simulink library "sl_nmea"  (R2017b)
settings: Solver=VariableStepAuto  StartTime=0.0  StopTime=10.0  RelTol=1e-3
settings Model: Creator=Bre  LastModifiedBy=bb6223s

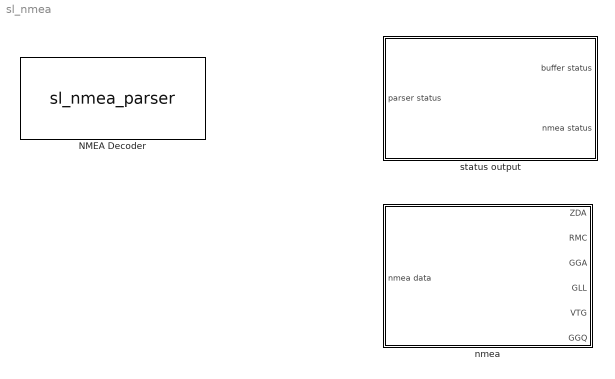
== system sl_nmea ==
  NMEA Decoder : S-Function  FunctionName=sl_nmea_parser  SFunctionModules='nmea0183 circularbuffer'  SFunctionDeploymentMode=off  EnableBusSupport=off  mask(NMEA Decoder){}
      mask help: NMEA message parser
      mask Display:
      | port_label('output',1,'status output')
      | port_label('output',2,'nmea output')
      | port_label('input',1,'data bytes')
      | port_label('input',2,'num data bytes')
      | color('brown');disp('{\bfgnss parser}', 'texmode', 'on')
  nmea : Subsystem
  status output : Subsystem

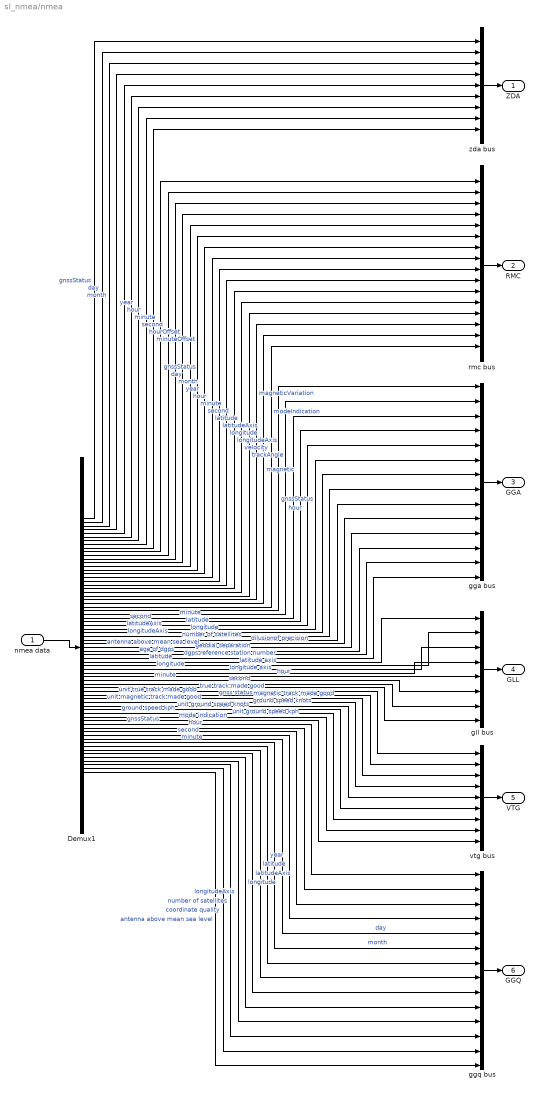
== system sl_nmea/nmea ==
  nmea data : Inport
  Demux1 : Demux  Outputs=70
  gga bus : BusCreator  Inputs=14
  ggq bus : BusCreator  Inputs=14
  gll bus : BusCreator  Inputs=8
  rmc bus : BusCreator  Inputs=16
  vtg bus : BusCreator  Inputs=9
  zda bus : BusCreator  Inputs=9
  ZDA : Outport
  RMC : Outport  Port=2
  GGA : Outport  Port=3
  GLL : Outport  Port=4
  VTG : Outport  Port=5
  GGQ : Outport  Port=6
  wires:
  Demux1/70 -> ggq bus/14  "antenna above mean sea level"
  Demux1/69 -> ggq bus/13  "coordinate quality"
  Demux1/68 -> ggq bus/12  "number of satellites"
  Demux1/67 -> ggq bus/11  "longitudeAxis"
  Demux1/66 -> ggq bus/10  "longitude"
  Demux1/65 -> ggq bus/9  "latitudeAxis"
  Demux1/64 -> ggq bus/8  "latitude"
  Demux1/63 -> ggq bus/7  "year"
  Demux1/62 -> ggq bus/6  "month"
  Demux1/61 -> ggq bus/5  "day"
  Demux1/60 -> ggq bus/4  "second"
  Demux1/59 -> ggq bus/3  "minute"
  Demux1/58 -> ggq bus/2  "hour"
  Demux1/57 -> ggq bus/1  "gnssStatus"
  ggq bus/1 -> GGQ/1
  Demux1/56 -> vtg bus/9  "mode indication"
  Demux1/55 -> vtg bus/8  "unit ground speed kph"
  Demux1/54 -> vtg bus/7  "ground speed kph"
  Demux1/53 -> vtg bus/6  "unit ground speed knots"
  Demux1/52 -> vtg bus/5  "ground speed knots"
  Demux1/51 -> vtg bus/4  "unit magnetic track made good"
  Demux1/50 -> vtg bus/3  "magnetic track made good"
  Demux1/49 -> vtg bus/2  "unit true track made good"
  Demux1/48 -> vtg bus/1  "true track made good"
  Demux1/47 -> gll bus/8  "gnss status"
  Demux1/46 -> gll bus/7  "second"
  Demux1/45 -> gll bus/6  "minute"
  Demux1/44 -> gll bus/5  "hour"
  Demux1/43 -> gll bus/4  "longitude axis"
  Demux1/42 -> gll bus/3  "longitude"
  Demux1/41 -> gll bus/2  "latitude axis"
  Demux1/40 -> gll bus/1  "latitude"
  vtg bus/1 -> VTG/1
  gll bus/1 -> GLL/1
  Demux1/39 -> gga bus/14  "dgps reference station number"
  Demux1/38 -> gga bus/13  "age of dgps"
  Demux1/37 -> gga bus/12  "geodial separation"
  Demux1/36 -> gga bus/11  "antenna above mean sea level"
  Demux1/35 -> gga bus/10  "dilusionof precision"
  Demux1/34 -> gga bus/9  "number of satellites"
  Demux1/33 -> gga bus/8  "longitudeAxis"
  Demux1/32 -> gga bus/7  "longitude"
  Demux1/31 -> gga bus/6  "latitudeAxis"
  Demux1/30 -> gga bus/5  "latitude"
  Demux1/29 -> gga bus/4  "second"
  Demux1/28 -> gga bus/3  "minute"
  Demux1/27 -> gga bus/2  "hour"
  Demux1/26 -> gga bus/1  "gnssStatus"
  gga bus/1 -> GGA/1
  Demux1/25 -> rmc bus/16  "modeIndication"
  Demux1/24 -> rmc bus/15  "magnetic"
  Demux1/23 -> rmc bus/14  "magneticVariation"
  Demux1/22 -> rmc bus/13  "trackAngle"
  Demux1/21 -> rmc bus/12  "velocity"
  Demux1/20 -> rmc bus/11  "longitudeAxis"
  Demux1/19 -> rmc bus/10  "longitude"
  Demux1/18 -> rmc bus/9  "latitudeAxis"
  Demux1/17 -> rmc bus/8  "latitude"
  Demux1/16 -> rmc bus/7  "second"
  Demux1/15 -> rmc bus/6  "minute"
  Demux1/14 -> rmc bus/5  "hour"
  Demux1/13 -> rmc bus/4  "year"
  Demux1/12 -> rmc bus/3  "month"
  Demux1/11 -> rmc bus/2  "day"
  Demux1/10 -> rmc bus/1  "gnssStatus"
  rmc bus/1 -> RMC/1
  Demux1/9 -> zda bus/9  "minuteOffset"
  Demux1/8 -> zda bus/8  "hourOffset"
  Demux1/7 -> zda bus/7  "second"
  Demux1/6 -> zda bus/6  "minute"
  Demux1/5 -> zda bus/5  "hour"
  Demux1/4 -> zda bus/4  "year"
  Demux1/3 -> zda bus/3  "month"
  Demux1/2 -> zda bus/2  "day"
  zda bus/1 -> ZDA/1
  nmea data/1 -> Demux1/1
  Demux1/1 -> zda bus/1  "gnssStatus"

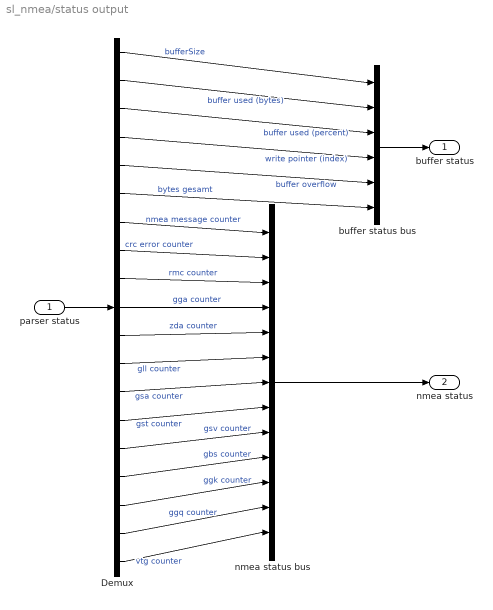
== system sl_nmea/status output ==
  parser status : Inport
  Demux : Demux  Outputs=19
  buffer status bus : BusCreator  Inputs=6
  nmea status bus : BusCreator  Inputs=13
  buffer status : Outport
  nmea status : Outport  Port=2
  wires:
  Demux/19 -> nmea status bus/13  "vtg counter"
  Demux/18 -> nmea status bus/12  "ggq counter"
  Demux/17 -> nmea status bus/11  "ggk counter"
  nmea status bus/1 -> nmea status/1
  buffer status bus/1 -> buffer status/1
  Demux/16 -> nmea status bus/10  "gbs counter"
  Demux/15 -> nmea status bus/9  "gsv counter"
  Demux/14 -> nmea status bus/8  "gst counter"
  Demux/13 -> nmea status bus/7  "gsa counter"
  Demux/12 -> nmea status bus/6  "gll counter"
  Demux/11 -> nmea status bus/5  "zda counter"
  Demux/10 -> nmea status bus/4  "gga counter"
  Demux/9 -> nmea status bus/3  "rmc counter"
  Demux/8 -> nmea status bus/2  "crc error counter"
  Demux/7 -> nmea status bus/1  "nmea message counter"
  Demux/6 -> buffer status bus/6  "bytes gesamt"
  Demux/5 -> buffer status bus/5  "buffer overflow"
  Demux/4 -> buffer status bus/4  "write pointer (index)"
  Demux/3 -> buffer status bus/3  "buffer used (percent)"
  Demux/2 -> buffer status bus/2  "buffer used (bytes)"
  parser status/1 -> Demux/1
  Demux/1 -> buffer status bus/1  "bufferSize"
